simulink model "vertical_smm_with_lqr_2d"  (R2014b)
settings: Solver=FixedStepDiscrete  StartTime=0.0  StopTime=inf  FixedStep=sample_time  RelTol=1e-3
values from neighbouring files (symbols this model uses):
  forward_dx = [-0.304875592207 -0.274388032987 -0.243900473766 -0.213412914545 -0.182925355324 -0.152437796104 -0.121950236883 -0.0914626776622 -0.0609751184415 -0.0304875592207 0 0.0304875592207 ... (714 elements, 21x34)]    [ref_trajs.mat]
  forward_dx_of_dxstar = [-1.3048755994 -1.25487559904 -1.20487559868 -1.15487559832 -1.10487559796 -1.0548755976 -1.00487559724 -0.954875596883 -0.904875596523 -0.854875596164 -0.804875595804 -0.754875595707 ... (29274 elements, 41x21x34)]    [ref_trajs.mat]
  forward_x = [0.0961104217981 0.0864993796183 0.0768883374385 0.0672772952586 0.0576662530788 0.048055210899 0.0384441687192 0.0288331265394 0.0192220843596 0.00961104217981 0 -0.00961104217981 ... (714 elements, 21x34)]    [ref_trajs.mat]
  forward_x_of_dxstar = [0.247353819189 0.239791649319 0.232229479449 0.22466730958 0.21710513971 0.209542969841 0.201980799971 0.194418630102 0.186856460232 0.179294290363 0.171732120493 0.164169950675 ... (29274 elements, 41x21x34)]    [ref_trajs.mat]
  target_dx_range = [-1 -0.95 -0.9 -0.85 -0.8 -0.75 -0.7 -0.65 -0.6 -0.55 -0.5 -0.45 ... (41 elements, 1x41)]    [ref_trajs.mat]
undefined symbols (not defined in the file or in its folder): A_kalman_fourbar_gear, A_kalman_transverse, A_kalman_vertical, A_lpf_dtau, A_lpf_leg_spring, B1_lpf_dtau, B1_lpf_leg_spring, B2_lpf_dtau, B2_lpf_leg_spring, B_dx_versus_x0, B_kalman_fourbar_gear, B_kalman_transverse, B_kalman_vertical, backwards_K_sag_of_t, boom_mount_angle, C_kalman_fourbar_gear, C_kalman_transverse, C_kalman_vertical, com_leg_motor, com_torso, contact_threshold, control_start_time, d_vertical_boom_com_offset, d_vertical_com, desired_com_forward_velocity, desired_torso_angle, Discrete, fcut_contact, forward_velocity_target_step, g, h_boom, HIP_MTR_MAX_CONT_TORQUE, i_robot, initial_dx_estimate, initial_dy_estimate, initial_dz_estimate, initial_z_estimate, j_leg, j_motor, j_segments, k_LQR_vertical, k_sea, k_vertical_winch, kalman_load_to_deflect_transmission, kalman_stance_slip_threshold, kd_lateral, kd_motor, kp_lateral, kp_motor, l_boom_projected, l_retract_delta, l_retract_swing_max, l_retract_swing_min, l_seg, lambda1, lambda2, lateral_offset, lateral_target_angle_right, lateral_transition_force, left_leg_flight_y_target ... (+55)
libraries: simulink x9, ctrlSharedLib x7
(part 3 of 4)

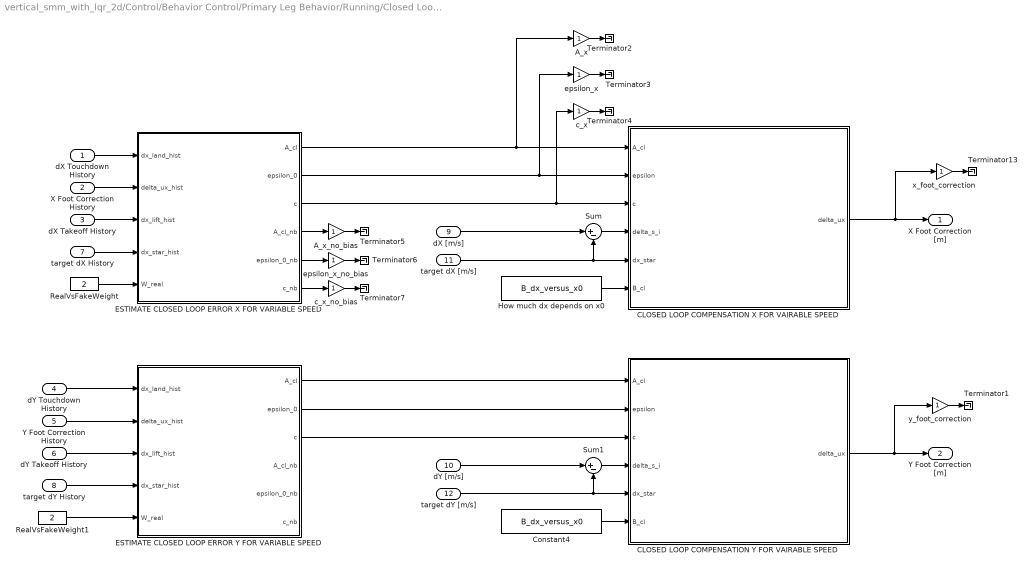
== system vertical_smm_with_lqr_2d/Control/Behavior Control/Primary Leg Behavior/Running/Closed Loop Compensation ==
  dX Touchdown History : Inport
  X Foot Correction History : Inport  Port=2
  dX Takeoff History : Inport  Port=3
  dY Touchdown History : Inport  Port=4
  Y Foot Correction History : Inport  Port=5
  dY Takeoff History : Inport  Port=6
  target dX History : Inport  Port=7
  target dY History : Inport  Port=8
  dX [m/s] : Inport  Port=9
  dY [m/s] : Inport  Port=10
  target dX [m/s] : Inport  Port=11
  "target dY [m/s] " : Inport  Port=12
  A_x : Gain
  A_x_no_bias : Gain
  CLOSED LOOP COMPENSATION X FOR VAIRABLE SPEED : MATLAB Function  TreatAsAtomicUnit=on
  CLOSED LOOP COMPENSATION Y FOR VAIRABLE SPEED : MATLAB Function  TreatAsAtomicUnit=on
  Constant4 : Constant  Value=B_dx_versus_x0
  ESTIMATE CLOSED LOOP ERROR X FOR VARIABLE SPEED : MATLAB Function  TreatAsAtomicUnit=on
  ESTIMATE CLOSED LOOP ERROR Y FOR VARIABLE SPEED : MATLAB Function  TreatAsAtomicUnit=on
  How much dx depends on x0 : Constant  Value=B_dx_versus_x0
  RealVsFakeWeight : Constant  Value=2
  RealVsFakeWeight1 : Constant  Value=2
  Sum : Sum  Inputs=|+-
  Sum1 : Sum  Inputs=|+-
  Terminator{1..7,13} (8 alike) : Terminator
  c_x : Gain
  c_x_no_bias : Gain
  epsilon_x : Gain
  epsilon_x_no_bias : Gain
  x_foot_correction : Gain
  y_foot_correction : Gain
  X Foot Correction [m] : Outport
  Y Foot Correction [m] : Outport  Port=2
  wires:
  RealVsFakeWeight1/1 -> ESTIMATE CLOSED LOOP ERROR Y FOR VARIABLE SPEED/5(W_real)
  Constant4/1 -> CLOSED LOOP COMPENSATION Y FOR VAIRABLE SPEED/6(B_cl)
  "target dY [m/s] "/1 -> Sum1/2, CLOSED LOOP COMPENSATION Y FOR VAIRABLE SPEED/5(dx_star)
  ESTIMATE CLOSED LOOP ERROR Y FOR VARIABLE SPEED/3(c) -> CLOSED LOOP COMPENSATION Y FOR VAIRABLE SPEED/3(c)
  ESTIMATE CLOSED LOOP ERROR Y FOR VARIABLE SPEED/2(epsilon_0) -> CLOSED LOOP COMPENSATION Y FOR VAIRABLE SPEED/2(epsilon)
  ESTIMATE CLOSED LOOP ERROR Y FOR VARIABLE SPEED/1(A_cl) -> CLOSED LOOP COMPENSATION Y FOR VAIRABLE SPEED/1(A_cl)
  target dY History/1 -> ESTIMATE CLOSED LOOP ERROR Y FOR VARIABLE SPEED/4(dx_star_hist)
  Y Foot Correction History/1 -> ESTIMATE CLOSED LOOP ERROR Y FOR VARIABLE SPEED/2(delta_ux_hist)
  dY Takeoff History/1 -> ESTIMATE CLOSED LOOP ERROR Y FOR VARIABLE SPEED/3(dx_lift_hist)
  dY [m/s]/1 -> Sum1/1
  RealVsFakeWeight/1 -> ESTIMATE CLOSED LOOP ERROR X FOR VARIABLE SPEED/5(W_real)
  How much dx depends on x0/1 -> CLOSED LOOP COMPENSATION X FOR VAIRABLE SPEED/6(B_cl)
  Sum/1 -> CLOSED LOOP COMPENSATION X FOR VAIRABLE SPEED/4(delta_s_i)
  target dX [m/s]/1 -> Sum/2, CLOSED LOOP COMPENSATION X FOR VAIRABLE SPEED/5(dx_star)
  ESTIMATE CLOSED LOOP ERROR X FOR VARIABLE SPEED/3(c) -> CLOSED LOOP COMPENSATION X FOR VAIRABLE SPEED/3(c), c_x/1
  ESTIMATE CLOSED LOOP ERROR X FOR VARIABLE SPEED/2(epsilon_0) -> CLOSED LOOP COMPENSATION X FOR VAIRABLE SPEED/2(epsilon), epsilon_x/1
  ESTIMATE CLOSED LOOP ERROR X FOR VARIABLE SPEED/1(A_cl) -> CLOSED LOOP COMPENSATION X FOR VAIRABLE SPEED/1(A_cl), A_x/1
  target dX History/1 -> ESTIMATE CLOSED LOOP ERROR X FOR VARIABLE SPEED/4(dx_star_hist)
  X Foot Correction History/1 -> ESTIMATE CLOSED LOOP ERROR X FOR VARIABLE SPEED/2(delta_ux_hist)
  dX Takeoff History/1 -> ESTIMATE CLOSED LOOP ERROR X FOR VARIABLE SPEED/3(dx_lift_hist)
  dX Touchdown History/1 -> ESTIMATE CLOSED LOOP ERROR X FOR VARIABLE SPEED/1(dx_land_hist)
  dX [m/s]/1 -> Sum/1
  dY Touchdown History/1 -> ESTIMATE CLOSED LOOP ERROR Y FOR VARIABLE SPEED/1(dx_land_hist)
  Sum1/1 -> CLOSED LOOP COMPENSATION Y FOR VAIRABLE SPEED/4(delta_s_i)
  CLOSED LOOP COMPENSATION X FOR VAIRABLE SPEED/1(delta_ux) -> x_foot_correction/1, X Foot Correction [m]/1
  x_foot_correction/1 -> Terminator13/1
  CLOSED LOOP COMPENSATION Y FOR VAIRABLE SPEED/1(delta_ux) -> y_foot_correction/1, Y Foot Correction [m]/1
  y_foot_correction/1 -> Terminator1/1
  A_x/1 -> Terminator2/1
  epsilon_x/1 -> Terminator3/1
  c_x/1 -> Terminator4/1
  ESTIMATE CLOSED LOOP ERROR X FOR VARIABLE SPEED/6(c_nb) -> c_x_no_bias/1
  ESTIMATE CLOSED LOOP ERROR X FOR VARIABLE SPEED/5(epsilon_0_nb) -> epsilon_x_no_bias/1
  ESTIMATE CLOSED LOOP ERROR X FOR VARIABLE SPEED/4(A_cl_nb) -> A_x_no_bias/1
  A_x_no_bias/1 -> Terminator5/1
  epsilon_x_no_bias/1 -> Terminator6/1
  c_x_no_bias/1 -> Terminator7/1

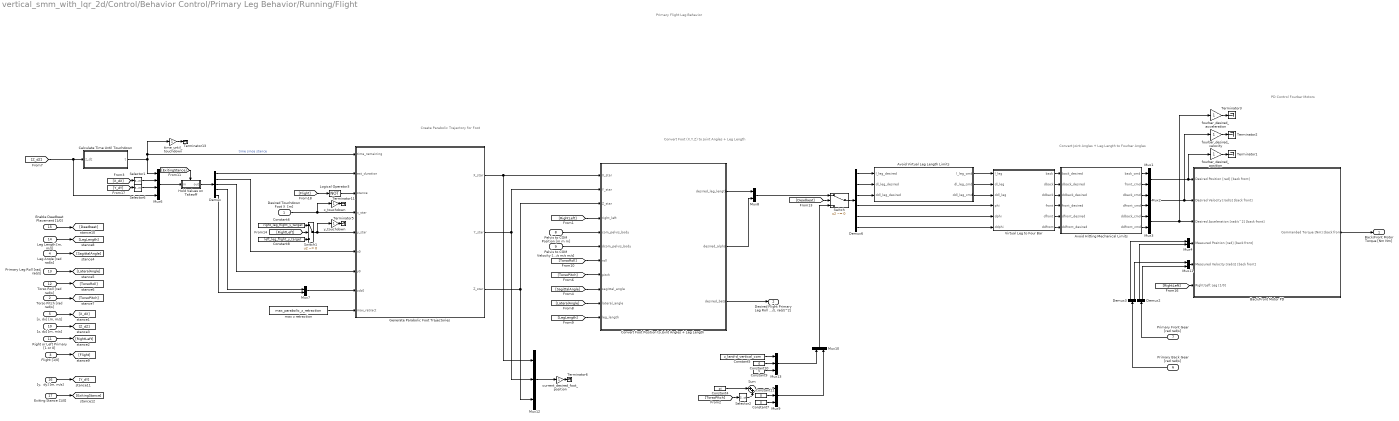
== system vertical_smm_with_lqr_2d/Control/Behavior Control/Primary Leg Behavior/Running/Flight ==
  note: Primary Flight Leg Behavior
  note: Create Parabolic
      | Trajectory for Foot
  note: Convert Foot (X,Y,Z) to
      | Joint Angles + Leg Length
  note: Convert Joint Angles + Leg Length
      | to Fourbar Angles
  note: PD Control Fourbar Motors
  Desired Touchdown Foot X  [m] : Inport
  Torso Pitch [rad rad/s] : Inport  Port=2
  Flight [1/0] : Inport  Port=3
  Leg Angle [rad rad/s] : Inport  Port=4
  "[x, dx] [m, m/s]" : Inport  Port=5
  Primary Back Gear [rad rad/s] : Inport  Port=6
  Primary Front Gear [rad rad/s] : Inport  Port=7
  Pelvis to COM Position [m m m] : Inport  Port=8
  Pelvis to COM Velocity [m/s m/s m/s] : Inport  Port=9
  "[z, dz] [m, m/s]" : Inport  Port=10
  Right or Left Primary [1 or 0] : Inport  Port=11
  Torso Roll [rad rad/s] : Inport  Port=12
  "Primary Leg Roll [rad, rad/s]" : Inport  Port=13
  "Leg Length [m, m/s]" : Inport  Port=14
  Enable Deadbeat Placement [1/0] : Inport  Port=15
  "[y,  dy] [m, m/s]" : Inport  Port=16
  Exiting Stance [1/0] : Inport  Port=17
  Avoid Hitting Mechanical Limits : MATLAB Function  TreatAsAtomicUnit=on
  Avoid Virtual Leg Length Limits : MATLAB Function  TreatAsAtomicUnit=on
  Back/Front Motor PD : Subsystem
  Calculate Time Until Touchdown : MATLAB Function  TreatAsAtomicUnit=on
  Constant{7,9..11} (4 alike) : Constant  Value=0
  Constant4 : Constant  Value=pi
  Constant5 : Constant  Value=z_land-d_vertical_com
  Constant6 : Constant  Value=right_leg_flight_y_target
  Constant8 : Constant  Value=left_leg_flight_y_target
  "Convert Foot Position to Joint Angles + Leg Length " : MATLAB Function  TreatAsAtomicUnit=on
  Demux : Demux  Outputs=5
  Demux2 : Demux  Outputs=2
  Demux3 : Demux  Outputs=2
  Demux6 : Demux  Outputs=6
  Generate Parabolic Foot Trajectories : MATLAB Function  TreatAsAtomicUnit=on
  Hold Values on Takeoff : Subsystem
  Logical Operator3 : Logic  Operator=NOT  AllPortsSameDT=off  OutDataTypeStr=boolean
  Mux{1..4,7..8,10..11} (8 alike) : Mux  Inputs=2
  Mux12 : Mux  Inputs=3
  Mux13 : Mux  Inputs=3
  Mux6 : Mux
  Mux9 : Mux  Inputs=3
  Selector1 : Selector  InputPortWidth=2  Indices=[1]
  Selector2 : Selector  InputPortWidth=2  Indices=[1]
  Selector6 : Selector  InputPortWidth=2  Indices=[1]
  Sum : Sum  Inputs=|++
  Switch : Switch  Criteria=u2 ~= 0
  Switch1 : Switch  Criteria=u2 ~= 0
  Terminator{1..3,5..6,11,13} (7 alike) : Terminator
  Virtual Leg to Four Bar : MATLAB Function  TreatAsAtomicUnit=on
  current_desired_foot_position : Gain
  fourbar_desired_acceleration : Gain
  fourbar_desired_position : Gain
  fourbar_desired_velocity : Gain
  max z retraction : Constant  Value=max_parabolic_z_retraction
  time_until_touchdown : Gain
  x_touchdown : Gain
  y_touchdown : Gain
  Back/Front Motor Torque [Nm Nm] : Outport
  "Desired Flight Primary Leg Roll [rad, rad/s, rad/s^2]" : Outport  Port=2
  wires:
  Virtual Leg to Four Bar/1(back) -> Avoid Hitting Mechanical Limits/1(back_desired)
  Virtual Leg to Four Bar/2(dback) -> Avoid Hitting Mechanical Limits/2(dback_desired)
  Virtual Leg to Four Bar/3(ddback) -> Avoid Hitting Mechanical Limits/3(ddback_desired)
  Virtual Leg to Four Bar/4(front) -> Avoid Hitting Mechanical Limits/4(front_desired)
  Virtual Leg to Four Bar/5(dfront) -> Avoid Hitting Mechanical Limits/5(dfront_desired)
  Virtual Leg to Four Bar/6(ddfront) -> Avoid Hitting Mechanical Limits/6(ddfront_desired)
  Mux11/1 -> Back/Front Motor PD/5(Measured Velocity [rad/s] [back front])
  Demux2/2 -> Mux11/2
  Mux4/1 -> Back/Front Motor PD/4(Measured Position [rad] [back front])
  Mux1/1 -> fourbar_desired_position/1, Back/Front Motor PD/1(Desired Position [rad] [back front])
  Demux3/2 -> Mux11/1
  Demux3/1 -> Mux4/1
  Avoid Hitting Mechanical Limits/2(front_cmd) -> Mux1/2
  Avoid Hitting Mechanical Limits/1(back_cmd) -> Mux1/1
  Demux2/1 -> Mux4/2
  Avoid Hitting Mechanical Limits/3(dback_cmd) -> Mux2/1
  Avoid Hitting Mechanical Limits/4(dfront_cmd) -> Mux2/2
  Avoid Hitting Mechanical Limits/5(ddback_cmd) -> Mux3/1
  Avoid Hitting Mechanical Limits/6(ddfront_cmd) -> Mux3/2
  Mux2/1 -> fourbar_desired_velocity/1, Back/Front Motor PD/2(Desired Velocity [rad/s] [back front])
  Mux3/1 -> fourbar_desired_acceleration/1, Back/Front Motor PD/3(Desired Acceleration [rad/s^2] [back front])
  Back/Front Motor PD/1(Commanded Torque [Nm] [back front]) -> Back/Front Motor Torque [Nm Nm]/1
  Primary Back Gear [rad rad/s]/1 -> Demux3/1
  Primary Front Gear [rad rad/s]/1 -> Demux2/1
  [RightLeft] -> Back/Front Motor PD/6(Right/Left Leg [1/0])
  fourbar_desired_position/1 -> Terminator1/1
  fourbar_desired_velocity/1 -> Terminator2/1
  fourbar_desired_acceleration/1 -> Terminator3/1
  Demux/1 -> Generate Parabolic Foot Trajectories/2(est_duration)
  Mux7/1 -> Generate Parabolic Foot Trajectories/8(zdz0)
  max z retraction/1 -> Generate Parabolic Foot Trajectories/9(max_retract)
  Logical Operator3/1 -> Generate Parabolic Foot Trajectories/3(stance)
  Mux6/1 -> Hold Values on Takeoff/1(in)
  Hold Values on Takeoff/1(out) -> Demux/1
  Switch1/1 -> Generate Parabolic Foot Trajectories/5(y_star), y_touchdown/1
  Selector1/1 -> Mux6/2
  [X_dX] -> Selector1/1
  Generate Parabolic Foot Trajectories/1(X_star) -> "Convert Foot Position to Joint Angles + Leg Length "/1(X_star), Mux12/1
  Generate Parabolic Foot Trajectories/2(Y_star) -> "Convert Foot Position to Joint Angles + Leg Length "/2(Y_star), Mux12/2
  Generate Parabolic Foot Trajectories/3(Z_star) -> "Convert Foot Position to Joint Angles + Leg Length "/3(Z_star), Mux12/3
  [RightLeft] -> "Convert Foot Position to Joint Angles + Leg Length "/4(right_left)
  "Convert Foot Position to Joint Angles + Leg Length "/2(desired_alpha) -> Mux8/2
  "Convert Foot Position to Joint Angles + Leg Length "/1(desired_leg_length) -> Mux8/1
  "Convert Foot Position to Joint Angles + Leg Length "/3(desired_beta) -> "Desired Flight Primary Leg Roll [rad, rad/s, rad/s^2]"/1
  Demux6/6 -> Virtual Leg to Four Bar/6(ddphi)
  Demux6/5 -> Virtual Leg to Four Bar/5(dphi)
  Demux6/4 -> Virtual Leg to Four Bar/4(phi)
  Switch/1 -> Demux6/1
  Mux8/1 -> Switch/1
  Constant7/1 -> Mux9/3
  Mux10/1 -> Switch/3
  Mux9/1 -> Mux10/2
  Leg Angle [rad rad/s]/1 -> [SagittalAngle]
  [SagittalAngle] -> "Convert Foot Position to Joint Angles + Leg Length "/9(sagittal_angle)
  Torso Pitch [rad rad/s]/1 -> [TorsoPitch]
  [TorsoPitch] -> "Convert Foot Position to Joint Angles + Leg Length "/8(pitch)
  [LateralAngle] -> "Convert Foot Position to Joint Angles + Leg Length "/10(lateral_angle)
  [LegLength] -> "Convert Foot Position to Joint Angles + Leg Length "/11(leg_length)
  [TorsoRoll] -> "Convert Foot Position to Joint Angles + Leg Length "/7(roll)
  Pelvis to COM Position [m m m]/1 -> "Convert Foot Position to Joint Angles + Leg Length "/5(com_pelvis_body)
  Pelvis to COM Velocity [m/s m/s m/s]/1 -> "Convert Foot Position to Joint Angles + Leg Length "/6(dcom_pelvis_body)
  Flight [1/0]/1 -> [Flight]
  [ExitingStance] -> Hold Values on Takeoff/Trigger
  [Deadbeat] -> Switch/2
  [RightLeft] -> Switch1/2
  Constant6/1 -> Switch1/1
  Constant8/1 -> Switch1/3
  "[x, dx] [m, m/s]"/1 -> [X_dX]
  Right or Left Primary [1 or 0]/1 -> [RightLeft]
  Torso Roll [rad rad/s]/1 -> [TorsoRoll]
  "Primary Leg Roll [rad, rad/s]"/1 -> [LateralAngle]
  "Leg Length [m, m/s]"/1 -> [LegLength]
  Enable Deadbeat Placement [1/0]/1 -> [Deadbeat]
  "[z, dz] [m, m/s]"/1 -> [Z_dZ]
  Desired Touchdown Foot X  [m]/1 -> x_touchdown/1, Generate Parabolic Foot Trajectories/4(x_star)
  x_touchdown/1 -> Terminator11/1
  y_touchdown/1 -> Terminator5/1
  current_desired_foot_position/1 -> Terminator6/1
  Mux12/1 -> current_desired_foot_position/1
  "[y,  dy] [m, m/s]"/1 -> [Y_dY]
  [Y_dY] -> Selector6/1
  [Z_dZ] -> Mux6/4, Calculate Time Until Touchdown/1(z_dz)
  Selector6/1 -> Mux6/3
  Demux/2 -> Generate Parabolic Foot Trajectories/6(x0)
  Demux/3 -> Generate Parabolic Foot Trajectories/7(y0)
  Demux/4 -> Mux7/1
  Demux/5 -> Mux7/2
  Calculate Time Until Touchdown/1(t) -> Mux6/1, time_until_touchdown/1, Generate Parabolic Foot Trajectories/1(time_remaining)  "time since stance"
  time_until_touchdown/1 -> Terminator13/1
  [Flight] -> Logical Operator3/1
  Constant11/1 -> Mux9/2
  Sum/1 -> Mux9/1
  Constant5/1 -> Mux13/1
  Constant9/1 -> Mux13/3
  Constant10/1 -> Mux13/2
  Mux13/1 -> Mux10/1
  Avoid Virtual Leg Length Limits/1(l_leg_cmd) -> Virtual Leg to Four Bar/1(l_leg)
  Avoid Virtual Leg Length Limits/2(dl_leg_cmd) -> Virtual Leg to Four Bar/2(dl_leg)
  Avoid Virtual Leg Length Limits/3(ddl_leg_cmd) -> Virtual Leg to Four Bar/3(ddl_leg)
  Demux6/1 -> Avoid Virtual Leg Length Limits/1(l_leg_desired)
  Demux6/2 -> Avoid Virtual Leg Length Limits/2(dl_leg_desired)
  Demux6/3 -> Avoid Virtual Leg Length Limits/3(ddl_leg_desired)
  Constant4/1 -> Sum/1
  [TorsoPitch] -> Selector2/1
  Selector2/1 -> Sum/2
  Exiting Stance [1/0]/1 -> [ExitingStance]

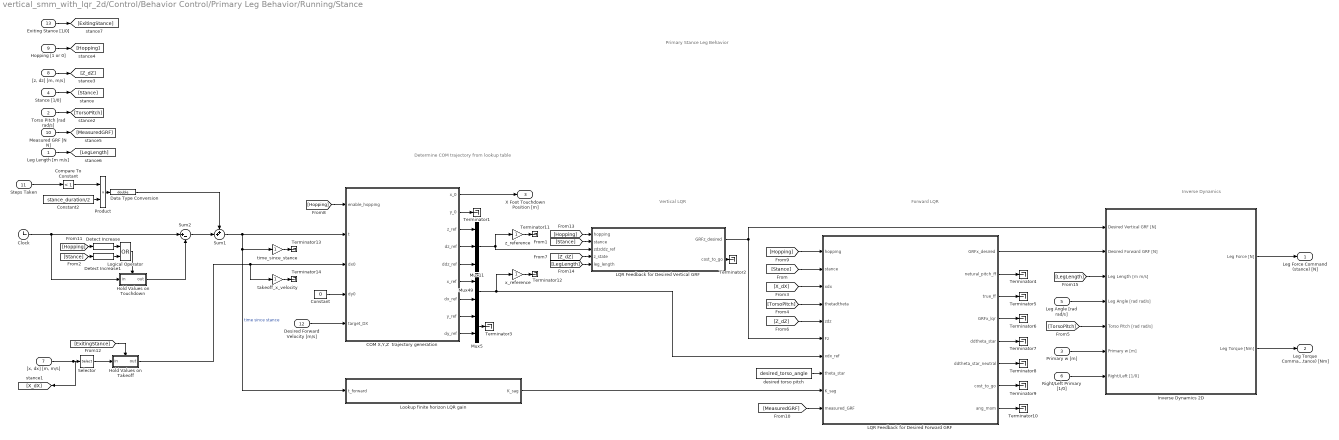
== system vertical_smm_with_lqr_2d/Control/Behavior Control/Primary Leg Behavior/Running/Stance ==
  note: Primary Stance Leg Behavior
  note: Determine COM trajectory
      | from lookup table
  note: Vertical LQR
  note: Forward LQR
  note: Inverse Dynamics
  Leg Length [m m/s] : Inport
  Torso Pitch [rad rad/s] : Inport  Port=2
  Primary w [m] : Inport  Port=3
  Stance [1/0] : Inport  Port=4
  Leg Angle [rad rad/s] : Inport  Port=5
  Right/Left Primary [1/0] : Inport  Port=6
  "[x, dx] [m, m/s]" : Inport  Port=7
  "[z, dz] [m, m/s]" : Inport  Port=8
  Hopping [1 or 0] : Inport  Port=9
  Measured GRF [N N] : Inport  Port=10
  Steps Taken : Inport  Port=11
  Desired Forward Velocity [m/s] : Inport  Port=12
  Exiting Stance [1/0] : Inport  Port=13
  COM X,Y,Z  trajectory generation : MATLAB Function  TreatAsAtomicUnit=on
  Clock : Clock
  Compare To Constant : simulink/Logic and Bit Operations/Compare To Constant  relop=<  const=1  OutDataTypeStr=uint8
  Constant : Constant  Value=0
  Constant2 : Constant  Value=stance_duration/2
  Data Type Conversion : DataTypeConversion  OutDataTypeStr=double
  Detect Increase : simulink/Logic and Bit Operations/Detect Increase  vinit=0.0  InputProcessing=Inherited  OutDataTypeStr=boolean
  Detect Increase1 : simulink/Logic and Bit Operations/Detect Increase  vinit=0.0  InputProcessing=Inherited  OutDataTypeStr=boolean
  Hold Values on Takeoff : Subsystem
  Hold Values on Touchdown : Subsystem
  Inverse Dynamics 2D : Subsystem
  LQR Feedback for Desired Forward GRF : MATLAB Function  TreatAsAtomicUnit=on
  LQR Feedback for Desired Vertical GRF : MATLAB Function  TreatAsAtomicUnit=on
  Logical Operator : Logic  Operator=OR  AllPortsSameDT=off  OutDataTypeStr=boolean
  Lookup finite horizon LQR gain : MATLAB Function  TreatAsAtomicUnit=on
  Mux11 : Mux  Inputs=3
  Mux49 : Mux  Inputs=2
  Mux5 : Mux  Inputs=2
  Product : Product
  Selector : Selector  InputPortWidth=2  Indices=[2]
  Sum1 : Sum  Inputs=++|  OutDataTypeStr=double
  Sum2 : Sum  Inputs=|+-
  Terminator{1..14} (14 alike) : Terminator
  desired torso pitch : Constant  Value=desired_torso_angle
  takeoff_x_velocity : Gain
  time_since_stance : Gain
  x_reference : Gain
  z_reference : Gain
  Leg Force Command (stance) [N] : Outport
  Leg Torque Command (stance) [Nm] : Outport  Port=2
  X Foot Touchdown Position [m] : Outport  Port=3
  wires:
  Inverse Dynamics 2D/2(Leg Torque [Nm]) -> Leg Torque Command (stance) [Nm]/1
  Inverse Dynamics 2D/1(Leg Force [N]) -> Leg Force Command (stance) [N]/1
  Mux5/1 -> Terminator3/1
  [Z_dZ] -> LQR Feedback for Desired Vertical GRF/4(z_state)
  COM X,Y,Z  trajectory generation/3(z_ref) -> Mux11/1
  [Stance] -> LQR Feedback for Desired Forward GRF/2(stance)
  COM X,Y,Z  trajectory generation/6(x_ref) -> Mux49/1
  COM X,Y,Z  trajectory generation/7(dx_ref) -> Mux49/2
  COM X,Y,Z  trajectory generation/8(y_ref) -> Mux5/1
  COM X,Y,Z  trajectory generation/9(dy_ref) -> Mux5/2
  COM X,Y,Z  trajectory generation/1(x_0) -> X Foot Touchdown Position [m]/1
  COM X,Y,Z  trajectory generation/4(dz_ref) -> Mux11/2
  COM X,Y,Z  trajectory generation/5(ddz_ref) -> Mux11/3
  Mux11/1 -> z_reference/1, LQR Feedback for Desired Vertical GRF/3(zdzddz_ref)
  [X_dX] -> LQR Feedback for Desired Forward GRF/3(xdx)
  [TorsoPitch] -> LQR Feedback for Desired Forward GRF/4(thetadtheta)
  Mux49/1 -> x_reference/1, LQR Feedback for Desired Forward GRF/7(xdx_ref)
  desired torso pitch/1 -> LQR Feedback for Desired Forward GRF/8(theta_star)
  Lookup finite horizon LQR gain/1(K_sag) -> LQR Feedback for Desired Forward GRF/9(K_sag)
  [Z_dZ] -> LQR Feedback for Desired Forward GRF/5(zdz)
  Desired Forward Velocity [m/s]/1 -> COM X,Y,Z  trajectory generation/5(target_DX)
  LQR Feedback for Desired Forward GRF/1(GRFx_desired) -> Inverse Dynamics 2D/2(Desired Forward GRF [N])
  Sum1/1 -> time_since_stance/1, Lookup finite horizon LQR gain/1(t_forward), COM X,Y,Z  trajectory generation/2(t)  "time since stance"
  LQR Feedback for Desired Vertical GRF/1(GRFz_desired) -> Inverse Dynamics 2D/1(Desired Vertical GRF [N]), LQR Feedback for Desired Forward GRF/6(Fz)
  Hold Values on Touchdown/1(out) -> Sum2/2
  Stance [1/0]/1 -> [Stance]
  [Stance] -> LQR Feedback for Desired Vertical GRF/2(stance)
  Logical Operator/1 -> Hold Values on Touchdown/Trigger
  "[x, dx] [m, m/s]"/1 -> [X_dX], Selector/1
  Clock/1 -> Hold Values on Touchdown/1(in), Sum2/1
  Constant/1 -> COM X,Y,Z  trajectory generation/4(dy0)
  LQR Feedback for Desired Vertical GRF/2(cost_to_go) -> Terminator2/1
  LQR Feedback for Desired Forward GRF/2(netural_pitch_ff) -> Terminator4/1
  LQR Feedback for Desired Forward GRF/3(true_ff) -> Terminator5/1
  LQR Feedback for Desired Forward GRF/4(GRFx_lqr) -> Terminator6/1
  LQR Feedback for Desired Forward GRF/5(ddtheta_star) -> Terminator7/1
  LQR Feedback for Desired Forward GRF/6(ddtheta_star_neutral) -> Terminator8/1
  LQR Feedback for Desired Forward GRF/7(cost_to_go) -> Terminator9/1
  LQR Feedback for Desired Forward GRF/8(ang_mom) -> Terminator10/1
  [LegLength] -> Inverse Dynamics 2D/3(Leg Length [m m/s])
  Leg Angle [rad rad/s]/1 -> Inverse Dynamics 2D/4(Leg Angle [rad rad/s])
  Torso Pitch [rad rad/s]/1 -> [TorsoPitch]
  [TorsoPitch] -> Inverse Dynamics 2D/5(Torso Pitch [rad rad/s])
  Primary w [m]/1 -> Inverse Dynamics 2D/6(Primary w [m])
  Right/Left Primary [1/0]/1 -> Inverse Dynamics 2D/7(Right/Left [1/0])
  "[z, dz] [m, m/s]"/1 -> [Z_dZ]
  COM X,Y,Z  trajectory generation/2(y_0) -> Terminator1/1
  Hopping [1 or 0]/1 -> [Hopping]
  [Hopping] -> COM X,Y,Z  trajectory generation/1(enable_hopping)
  z_reference/1 -> Terminator11/1
  x_reference/1 -> Terminator12/1
  [Hopping] -> LQR Feedback for Desired Forward GRF/1(hopping)
  Measured GRF [N N]/1 -> [MeasuredGRF]
  [MeasuredGRF] -> LQR Feedback for Desired Forward GRF/10(measured_GRF)
  Steps Taken/1 -> Compare To Constant/1
  Product/1 -> Data Type Conversion/1
  Constant2/1 -> Product/2
  Detect Increase/1 -> Logical Operator/1
  Detect Increase1/1 -> Logical Operator/2
  Compare To Constant/1 -> Product/1
  Sum2/1 -> Sum1/2
  Data Type Conversion/1 -> Sum1/1
  time_since_stance/1 -> Terminator13/1
  [Hopping] -> Detect Increase/1
  [Stance] -> Detect Increase1/1
  Hold Values on Takeoff/1(out) -> takeoff_x_velocity/1, COM X,Y,Z  trajectory generation/3(dx0)
  [ExitingStance] -> Hold Values on Takeoff/Trigger
  takeoff_x_velocity/1 -> Terminator14/1
  Selector/1 -> Hold Values on Takeoff/1(in)
  [Hopping] -> LQR Feedback for Desired Vertical GRF/1(hopping)
  [LegLength] -> LQR Feedback for Desired Vertical GRF/5(leg_length)
  Leg Length [m m/s]/1 -> [LegLength]
  Exiting Stance [1/0]/1 -> [ExitingStance]

== system vertical_smm_with_lqr_2d/Control/Behavior Control/Secondary Leg Behavior/Back//Front Motor PD/Friction Compensation ==
  Right/Left [1/0] : Inport
  Commanded Velocity [rad/s] [back front] : Inport  Port=2
  Product : Product
  Sign : Signum
  Sum1 : Sum
  Switch : Switch  Criteria=u2 ~= 0
  Switch1 : Switch  Criteria=u2 ~= 0
  coulomb_friction_left : Constant  Value=sea_coulomb_friction(3:4)
  coulomb_friction_right : Constant  Value=sea_coulomb_friction(1:2)
  offset_friction_left : Constant  Value=sea_offset_friction(3:4)
  offset_friction_right : Constant  Value=sea_offset_friction(1:2)
  Friction Compensation [Nm] : Outport
  wires:
  Commanded Velocity [rad/s] [back front]/1 -> Sign/1
  Switch/1 -> Sum1/2
  Sum1/1 -> Friction Compensation [Nm]/1
  Product/1 -> Sum1/1
  Right/Left [1/0]/1 -> Switch1/2, Switch/2
  offset_friction_right/1 -> Switch/1
  offset_friction_left/1 -> Switch/3
  coulomb_friction_right/1 -> Switch1/1
  coulomb_friction_left/1 -> Switch1/3
  Switch1/1 -> Product/2
  Sign/1 -> Product/1

== system vertical_smm_with_lqr_2d/Control/Behavior Control/Primary Leg Behavior/Running/Circular Buffer/Enabled on Touchdown ==
  In : Inport
  Enable : EnablePort
  Out : Outport
  wires:
  In/1 -> Out/1

== system vertical_smm_with_lqr_2d/Control/Behavior Control/Primary Leg Behavior/Running/Flight/Back//Front Motor PD ==
  Desired Position [rad] [back front] : Inport
  Desired Velocity [rad/s] [back front] : Inport  Port=2
  Desired Acceleration [rad/s^2] [back front] : Inport  Port=3
  Measured Position [rad] [back front] : Inport  Port=4
  Measured Velocity [rad/s] [back front] : Inport  Port=5
  Right/Left Leg [1/0] : Inport  Port=6
  Friction Compensation : Subsystem
  Product : Product
  Sum1 : Sum  Inputs=|++
  Sum2 : Sum  Inputs=|++
  Sum7 : Sum  Inputs=|+-
  Sum8 : Sum  Inputs=|+-
  Sum9 : Sum
  kd : Gain  Gain=kd_motor
  kp : Gain  Gain=kp_motor
  reflected inertia : Constant  Value=j_motor
  Commanded Torque [Nm] [back front] : Outport
  wires:
  kp/1 -> Sum9/1
  Sum7/1 -> kp/1
  Measured Position [rad] [back front]/1 -> Sum7/2
  Sum9/1 -> Sum1/1
  Sum8/1 -> kd/1
  Desired Position [rad] [back front]/1 -> Sum7/1
  kd/1 -> Sum9/2
  Measured Velocity [rad/s] [back front]/1 -> Sum8/2
  Sum1/1 -> Sum2/1
  Desired Acceleration [rad/s^2] [back front]/1 -> Product/1
  Product/1 -> Sum1/2
  Right/Left Leg [1/0]/1 -> Friction Compensation/1(Right/Left [1/0])
  Sum2/1 -> Commanded Torque [Nm] [back front]/1
  Desired Velocity [rad/s] [back front]/1 -> Friction Compensation/2(Commanded Velocity [rad/s] [back front]), Sum8/1
  reflected inertia/1 -> Product/2
  Friction Compensation/1(Friction Compensation [Nm]) -> Sum2/2

== system vertical_smm_with_lqr_2d/Control/Behavior Control/Primary Leg Behavior/Running/Flight/Hold Values on Takeoff ==
  in : Inport
  Trigger : TriggerPort  ShowOutputPort=on  PortDimensions=1
  Subsystem : Subsystem
  out : Outport
  wires:
  Trigger/1 -> Subsystem/Enable
  Subsystem/1(out) -> out/1
  in/1 -> Subsystem/1(in)

== system vertical_smm_with_lqr_2d/Control/Behavior Control/Primary Leg Behavior/Running/Stance/Hold Values on Takeoff ==
  in : Inport
  Trigger : TriggerPort  ShowOutputPort=on  PortDimensions=1
  Subsystem : Subsystem
  out : Outport
  wires:
  Trigger/1 -> Subsystem/Enable
  Subsystem/1(out) -> out/1
  in/1 -> Subsystem/1(in)

== system vertical_smm_with_lqr_2d/Control/Behavior Control/Primary Leg Behavior/Running/Stance/Hold Values on Touchdown ==
  in : Inport
  Trigger : TriggerPort  ShowOutputPort=on  PortDimensions=1
  Subsystem : Subsystem
  out : Outport
  wires:
  in/1 -> Subsystem/1(in)
  Subsystem/1(out) -> out/1
  Trigger/1 -> Subsystem/Enable

== system vertical_smm_with_lqr_2d/Control/Behavior Control/Primary Leg Behavior/Running/Stance/Inverse Dynamics 2D ==
  Desired Vertical GRF [N] : Inport
  Desired Forward GRF [N] : Inport  Port=2
  Leg Length [m m/s] : Inport  Port=3
  Leg Angle [rad rad/s] : Inport  Port=4
  Torso Pitch [rad rad/s] : Inport  Port=5
  Primary w [m] : Inport  Port=6
  Right/Left [1/0] : Inport  Port=7
  Constant2 : Constant  Value=0
  Demux5 : Demux  Outputs=2
  Leg Force-Torque Distribution : Subsystem
  Spring Torques : Selector  InputPortWidth=7  Indices=[6 7]
  Terminator1 : Terminator
  Terminator3 : Terminator
  desired_forward_GRF : Gain
  desired_vertical_GRF : Gain
  target_GRF_inverse_dynamics : MATLAB Function  TreatAsAtomicUnit=on
  Leg Force [N] : Outport
  Leg Torque [Nm] : Outport  Port=2
  wires:
  Leg Force-Torque Distribution/1(Leg Force [N]) -> Leg Force [N]/1
  Leg Angle [rad rad/s]/1 -> target_GRF_inverse_dynamics/5(phi)
  Torso Pitch [rad rad/s]/1 -> target_GRF_inverse_dynamics/4(theta)
  Leg Force-Torque Distribution/2(Leg Torque [Nm]) -> Leg Torque [Nm]/1
  Primary w [m]/1 -> Leg Force-Torque Distribution/3(w [m]), target_GRF_inverse_dynamics/7(w)
  Spring Torques/1 -> Demux5/1
  Demux5/1 -> Leg Force-Torque Distribution/1(Front Spring Torque [Nm])
  Demux5/2 -> Leg Force-Torque Distribution/2(Back Spring Torque [Nm])
  target_GRF_inverse_dynamics/1(z) -> Spring Torques/1
  Constant2/1 -> target_GRF_inverse_dynamics/9(tau_rotor_b), target_GRF_inverse_dynamics/8(tau_rotor_f)
  Leg Length [m m/s]/1 -> target_GRF_inverse_dynamics/6(l_leg)
  Right/Left [1/0]/1 -> target_GRF_inverse_dynamics/3(right_left)
  Desired Forward GRF [N]/1 -> desired_forward_GRF/1, target_GRF_inverse_dynamics/1(GRFx)
  desired_forward_GRF/1 -> Terminator3/1
  Desired Vertical GRF [N]/1 -> desired_vertical_GRF/1, target_GRF_inverse_dynamics/2(GRFz)
  desired_vertical_GRF/1 -> Terminator1/1

== system vertical_smm_with_lqr_2d/Control/Behavior Control/Primary Leg Behavior/Running/Flight/Back//Front Motor PD/Friction Compensation ==
  Right/Left [1/0] : Inport
  Commanded Velocity [rad/s] [back front] : Inport  Port=2
  Product : Product
  Sign : Signum
  Sum1 : Sum
  Switch : Switch  Criteria=u2 ~= 0
  Switch1 : Switch  Criteria=u2 ~= 0
  coulomb_friction_left : Constant  Value=sea_coulomb_friction(3:4)
  coulomb_friction_right : Constant  Value=sea_coulomb_friction(1:2)
  offset_friction_left : Constant  Value=sea_offset_friction(3:4)
  offset_friction_right : Constant  Value=sea_offset_friction(1:2)
  Friction Compensation [Nm] : Outport
  wires:
  Commanded Velocity [rad/s] [back front]/1 -> Sign/1
  Switch/1 -> Sum1/2
  Sum1/1 -> Friction Compensation [Nm]/1
  Product/1 -> Sum1/1
  Right/Left [1/0]/1 -> Switch1/2, Switch/2
  offset_friction_right/1 -> Switch/1
  offset_friction_left/1 -> Switch/3
  coulomb_friction_right/1 -> Switch1/1
  coulomb_friction_left/1 -> Switch1/3
  Switch1/1 -> Product/2
  Sign/1 -> Product/1

== system vertical_smm_with_lqr_2d/Control/Behavior Control/Primary Leg Behavior/Running/Flight/Hold Values on Takeoff/Subsystem ==
  in : Inport
  Enable : EnablePort
  out : Outport
  wires:
  in/1 -> out/1

== system vertical_smm_with_lqr_2d/Control/Behavior Control/Primary Leg Behavior/Running/Stance/Hold Values on Takeoff/Subsystem ==
  in : Inport
  Enable : EnablePort
  out : Outport
  wires:
  in/1 -> out/1

== system vertical_smm_with_lqr_2d/Control/Behavior Control/Primary Leg Behavior/Running/Stance/Hold Values on Touchdown/Subsystem ==
  in : Inport
  Enable : EnablePort
  out : Outport
  wires:
  in/1 -> out/1

== system vertical_smm_with_lqr_2d/Control/Behavior Control/Primary Leg Behavior/Running/Stance/Inverse Dynamics 2D/Leg Force-Torque Distribution ==
  Front Spring Torque [Nm] : Inport
  Back Spring Torque [Nm] : Inport  Port=2
  w [m] : Inport  Port=3
  Divide : Product  Inputs=*/
  Sum2 : Sum  Inputs=+|+
  Sum5 : Sum  Inputs=+|-
  Leg Force [N] : Outport
  Leg Torque [Nm] : Outport  Port=2
  wires:
  Sum2/1 -> Leg Torque [Nm]/1
  Back Spring Torque [Nm]/1 -> Sum5/2, Sum2/2
  Sum5/1 -> Divide/1
  w [m]/1 -> Divide/2
  Front Spring Torque [Nm]/1 -> Sum5/1, Sum2/1
  Divide/1 -> Leg Force [N]/1

== stateflow chart vertical_smm_with_lqr_2d/Control/Behavior Control/Primary Leg Behavior/State Machine ==
  state TouchDown
  state LockedContact
  state Unloading
  state Takeoff
  state Flight
  (junction 91) -> TouchDown
  TouchDown -> (junction 130) [order 2] : [vertical_grf < contact_threshold]
  (junction 93) -> (junction 91)
  (junction 130) -> (junction 128)
  TouchDown -> LockedContact [order 1] : [vertical_grf > loaded_threshold]
  (junction 115) -> LockedContact
  (junction 118) -> (junction 115)
  LockedContact -> Unloading : [leg_velocity >= 0 && previous_leg_velocity < 0]
  Unloading -> LockedContact [order 2] : [vertical_grf > loaded_threshold && leg_velocity < 0]
  (junction 122) -> (junction 118)
  Unloading -> Takeoff [order 1] : [vertical_grf < contact_threshold || leg_length > max_leg_length]
  Takeoff -> Flight : after(t_flight,sec)
  (default) -> Flight
  Flight -> (junction 93) : [vertical_grf > contact_threshold]
  (junction 128) -> Flight
  data: leg_length input; leg_velocity input; previous_leg_velocity input; vertical_grf input; t_flight parameter; max_leg_length parameter; contact_threshold parameter; loaded_threshold parameter; TouchDown output boolean; LockedContact output boolean; Unloading output boolean; Takeoff output boolean; Flight output boolean

== matlab function vertical_smm_with_lqr_2d/Control/Behavior Control/Primary Leg Behavior/Running/Stance/LQR Feedback for Desired Forward GRF ==
  data: hopping input; stance input; GRFx_desired output; netural_pitch_ff output; true_ff output; GRFx_lqr output; ddtheta_star output; ddtheta_star_neutral output; xdx input; thetadtheta input; zdz input; Fz input; xdx_ref input size=2; theta_star input; K_sag input; measured_GRF input; i_robot parameter; P_LQR_sagittal parameter; cost_to_go output double size=1; ang_mom output
%% LQR for x state

% stance: 1 if in stance, 0 otherwise
% xdx: [ x from stance leg to COM, dx of COM]
% thetadtheta: [pitch, dpitch]
% zdz: [z of COM, dz of COM]
% Fz: Desired z GRF
% xdx_ref: [x, dx] current reference point for COM
% theta_star: desired torso pitch
% K_sag: time dependent LQR gain


% sagittal_state: [x, pitch, dx, dptich]
% theta_star: desired torso pitch


function [GRFx_desired, netural_pitch_ff, true_ff, GRFx_lqr, ddtheta_star, ddtheta_star_neutral, cost_to_go, ang_mom]  =  ...
    LQR_Sagittal(hopping, stance, xdx, thetadtheta, zdz, Fz, xdx_ref, theta_star, K_sag, measured_GRF, i_robot,...
    P_LQR_sagittal)

    sagittal_state = [xdx(1); thetadtheta(1); xdx(2); thetadtheta(2)];
    sagittal_reference = [xdx_ref(1), theta_star, xdx_ref(2), 0]';
    
    % make the target pitch depend on current pitch rate s.t system ends at theta_star after flight
%     sagittal_reference = [xdx_ref(1), theta_star - f_duration*thetadtheta(2), xdx_ref(2), 0]';
    sagittal_error = (sagittal_state - sagittal_reference);
    
   
    GRFx_lqr = - K_sag*sagittal_error;
    cost_to_go = sagittal_error'*P_LQR_sagittal*sagittal_error;
    netural_pitch_ff = Fz*xdx(1)/zdz(1);
    true_ff = Fz*xdx_ref(1)/zdz(1);
    
    if stance == 0
      GRFx_lqr = 0;
      cost_to_go = 0;
      netural_pitch_ff = 0;
      true_ff = 0;
    end
    
    GRFx_desired = netural_pitch_ff + GRFx_lqr;
    %GRFx_desired = i_robot/zdz(1)*(-150*(theta_star-thetadtheta(1)) + 30*thetadtheta(2)) + netural_pitch_ff;
    if ~hopping % different PD law for lowering off the winch
        GRFx_desired = i_robot/zdz(1)*(-150*(theta_star-thetadtheta(1)) + 30*thetadtheta(2)) + netural_pitch_ff;
    end
    GRFx_desired = min(max(GRFx_desired, -abs(measured_GRF(2))/2), abs(measured_GRF(2))/2); % saturate to friction cone (mu = 0.5)
       
    % quantities for logging
    ddtheta_star_neutral = -(GRFx_lqr)*zdz(1)/i_robot;
    ddtheta_star = -(GRFx_desired - netural_pitch_ff)*zdz(1)/i_robot;
    ang_mom = i_robot*thetadtheta(2);
end

== matlab function vertical_smm_with_lqr_2d/Control/Behavior Control/Torque Distribution Right/Motor Torque Saturation Optimization ==
  data: x1s input; t1 output; x2s input; lambda1 parameter; lambda2 parameter; max_torque_sagittal parameter; t2 output
% Optimal leg motor torque distribution
function [t1, t2] = distribute_torque(x1s, x2s, lambda1, lambda2, max_torque_sagittal)

s = max_torque_sagittal;

% possible solutions
x1 = [                                                      x1s;
                                                            0;
                                                            s;
                                                            0;
                                                           -s;
  (lambda2*s + lambda1*x1s - lambda2*x2s)/(lambda1 + lambda2);
  (lambda1*x1s - lambda2*s + lambda2*x2s)/(lambda1 + lambda2);
  (lambda2*s + lambda1*x1s + lambda2*x2s)/(lambda1 + lambda2);
 -(lambda2*s - lambda1*x1s + lambda2*x2s)/(lambda1 + lambda2)];
 
x2 = [                                                      x2s;
                                                            s;
                                                            0;
                                                           -s;
                                                            0;
  (lambda1*s - lambda1*x1s + lambda2*x2s)/(lambda1 + lambda2);
  (lambda1*s + lambda1*x1s + lambda2*x2s)/(lambda1 + lambda2);
  (lambda1*x1s - lambda1*s + lambda2*x2s)/(lambda1 + lambda2);
 -(lambda1*s + lambda1*x1s - lambda2*x2s)/(lambda1 + lambda2)];

% test constraints
c1 = s - x1 - x2 >= 0;
c2 = s + x1 + x2 >= 0;
c3 = s - x1 + x2 >= 0;
c4 = s + x1 - x2 >= 0;
constraints = c1 & c2 & c3 & c4;

% objective function to maximize
f = -lambda1*(x1-x1s).^2-lambda2*(x2-x2s).^2;
satisfied = find(constraints);
[~,I] = max(f(satisfied));

t1 = x1(satisfied(I));
t2 = x2(satisfied(I));

== matlab function vertical_smm_with_lqr_2d/Control/Behavior Control/Secondary Leg Behavior/Avoid Hitting Mechanical Limits ==
  data: back_cmd output double; front_cmd output double; dback_cmd output double; dfront_cmd output double; ddback_cmd output double; ddfront_cmd output double; back_desired input; dback_desired input; ddback_desired input; front_desired input; dfront_desired input; ddfront_desired input; min_front_bar_angle parameter; max_front_bar_angle parameter; min_back_bar_angle parameter; max_back_bar_angle parameter
%% Avoid joint limits by ensuring we don't command velocities/accelerations that would push us into them when we are close to them.
function [back_cmd, front_cmd, dback_cmd, dfront_cmd, ddback_cmd, ddfront_cmd] ...
    = AvoidFourbarLimits(back_desired,dback_desired, ddback_desired, ...
          front_desired, dfront_desired, ddfront_desired, ...
          min_front_bar_angle, max_front_bar_angle, min_back_bar_angle, max_back_bar_angle)
    [back_cmd, front_cmd, dback_cmd, dfront_cmd, ddback_cmd, ddfront_cmd] = AvoidFourbarLimits(back_desired,dback_desired, ddback_desired, front_desired, dfront_desired, ddfront_desired, min_front_bar_angle, max_front_bar_angle, min_back_bar_angle, max_back_bar_angle);
end

== matlab function vertical_smm_with_lqr_2d/Control/Behavior Control/State Estimation/PositionUsingRobotGeometry ==
  data: right_left input; horizontal_com_position output; roll input; pitch input; yaw input; horizontal_com_velocity output; lateral_com_position output; lateral_com_velocity output; left_leg_sagittal_angle input; left_leg_lateral_angle input; left_leg_length input; right_leg_sagittal_angle input; right_leg_lateral_angle input; right_leg_length input; m_torso parameter; m_leg_motor parameter; m_leg parameter; com_torso parameter; com_leg_motor parameter; lateral_offset parameter; vertical_com_position output; vertical_com_velocity output; com_left_foot output; dcom_left_foot output; com_right_foot output; dcom_right_foot output; com_pelvis output; dcom_pelvis output
% Returns 2D COM relative to primary foot
function [horizontal_com_position, horizontal_com_velocity, ...
          lateral_com_position, lateral_com_velocity, ...
          vertical_com_position, vertical_com_velocity, ...
          com_left_foot, dcom_left_foot, com_right_foot, dcom_right_foot, ....
          com_pelvis, dcom_pelvis] = ...
         ComPositionUsingRobotGeometry(right_left, ...
                                    roll, pitch, yaw, ...
                                    left_leg_sagittal_angle, left_leg_lateral_angle, left_leg_length, ...
                                    right_leg_sagittal_angle, right_leg_lateral_angle, right_leg_length, ...
                                    m_torso, m_leg_motor, m_leg, com_torso, com_leg_motor, lateral_offset)
                    
    q =  [roll(1), pitch(1), yaw(1), left_leg_sagittal_angle(1), left_leg_lateral_angle(1), left_leg_length(1), right_leg_sagittal_angle(1), right_leg_lateral_angle(1), right_leg_length(1)];
    dq = [roll(2), pitch(2), yaw(2), left_leg_sagittal_angle(2), left_leg_lateral_angle(2), left_leg_length(2), right_leg_sagittal_angle(2), right_leg_lateral_angle(2), right_leg_length(2)];
                    
    [ com_pelvis, dcom_pelvis, ...
      com_left_foot, dcom_left_foot, ...
      com_right_foot, dcom_right_foot ] = ...
    ComCalculationFromRobot( q, dq, m_torso, m_leg_motor, m_leg, com_torso, com_leg_motor, lateral_offset );

    if right_left
        com_position = com_right_foot(4:6);
        com_velocity = dcom_right_foot(4:6);
    else
        com_position = com_left_foot(4:6);
        com_velocity = dcom_left_foot(4:6);
    end


    horizontal_com_position = com_position(1);
    horizontal_com_velocity = com_velocity(1);
    lateral_com_position = com_position(2);
    lateral_com_velocity = com_velocity(2);
    vertical_com_position = com_position(3);
    vertical_com_velocity = com_velocity(3);

end

== matlab function vertical_smm_with_lqr_2d/Control/Behavior Control/Torque Distribution Left/Motor Torque Saturation Optimization ==
  data: x1s input; t1 output; x2s input; lambda1 parameter; lambda2 parameter; max_torque_sagittal parameter; t2 output
% Optimal leg motor torque distribution
function [t1, t2] = distribute_torque(x1s, x2s, lambda1, lambda2, max_torque_sagittal)

s = max_torque_sagittal;

% possible solutions
x1 = [                                                      x1s;
                                                            0;
                                                            s;
                                                            0;
                                                           -s;
  (lambda2*s + lambda1*x1s - lambda2*x2s)/(lambda1 + lambda2);
  (lambda1*x1s - lambda2*s + lambda2*x2s)/(lambda1 + lambda2);
  (lambda2*s + lambda1*x1s + lambda2*x2s)/(lambda1 + lambda2);
 -(lambda2*s - lambda1*x1s + lambda2*x2s)/(lambda1 + lambda2)];
 
x2 = [                                                      x2s;
                                                            s;
                                                            0;
                                                           -s;
                                                            0;
  (lambda1*s - lambda1*x1s + lambda2*x2s)/(lambda1 + lambda2);
  (lambda1*s + lambda1*x1s + lambda2*x2s)/(lambda1 + lambda2);
  (lambda1*x1s - lambda1*s + lambda2*x2s)/(lambda1 + lambda2);
 -(lambda1*s + lambda1*x1s - lambda2*x2s)/(lambda1 + lambda2)];

% test constraints
c1 = s - x1 - x2 >= 0;
c2 = s + x1 + x2 >= 0;
c3 = s - x1 + x2 >= 0;
c4 = s + x1 - x2 >= 0;
constraints = c1 & c2 & c3 & c4;

% objective function to maximize
f = -lambda1*(x1-x1s).^2-lambda2*(x2-x2s).^2;
satisfied = find(constraints);
[~,I] = max(f(satisfied));

t1 = x1(satisfied(I));
t2 = x2(satisfied(I));

== matlab function vertical_smm_with_lqr_2d/Control/Behavior Control/State Estimation/Kalman Filtering/eigen values ==
  data: Z input; E output
function E = eigen(Z)
    E = real(eig(Z));
    E = sort(E);
end

== matlab function vertical_smm_with_lqr_2d/Control/Behavior Control/Primary Leg Behavior/Running/Flight/Generate Parabolic Foot Trajectories ==
  data: time_remaining input; est_duration input; stance input; x_star input; y_star input; x0 input; y0 input; zdz0 input; max_retract input; z_land parameter; min_f_duration parameter; X_star output size=3; Y_star output size=3; Z_star output size=3
%% Parabolic trajectory generation for x, y, and z
% est_duration: estimated flight time
% time_remaining: time until estimated touchdown
% stance: 1 if in stance, 0 otherwise
% x_star: desired x for foot to COM
% y_star: desired y for foot to COM
% x0: x position at takeoff
% y0: y position at takeoff
% zdz0: [z, dz] at takeoff
% max_retract: how high to lift z for ground clearance
% z_land: nominal z height for landing
% min_f_duration: minimum trajectory time

function [X_star, Y_star, Z_star]  =  ...
          GenerateParabolicFootTrajectory(time_remaining, est_duration,  ...
                               stance, x_star, y_star, x0, y0, zdz0, ...
                               max_retract,  z_land, min_f_duration)
% we are solving for yawed coordinates xyz of com-foot in flight and
% converting them to joint angles

% estimate z ballistically
% z = z_dz_liftoff(1) + z_dz_liftoff(2)*t_flight -g/2*t_flight^2;
% dz = z_dz_liftoff(2) - g*t_flight;
% 
% z = com_xdx_ydy_zdz(5); dz = com_xdx_ydy_zdz(6);
% time_remaining = (-dz-sqrt(max(dz^2 - 4*g/2*(z_land-z), 0) ) )/ (-g); % ballistic estimate of landing

% if stance || time_remaining < 0
if stance
  X_star = [0;0;0]; Y_star = [0;0;0]; Z_star = [z_land-max_retract;0;0];   
else
  % plan a traj from init to desired in estimated duration. Use a
  % discontinuous initial condition if estimated duration too short.
  duration = max(est_duration, min_f_duration);
  t_r = max(min(time_remaining, duration),0);
  % sweep a parabola from x0 to x_star with dx_end = 0
  x_star_t = x_star + (x0-x_star)*(t_r/duration)^2;
  dx_star_t = -(x0-x_star)*2*(t_r/duration)/duration;
  ddx_star_t = (x0-x_star)*2/duration^2;
  % same for y
  y_star_t = y_star + (y0-y_star)*(t_r/duration)^2;
  dy_star_t = -(y0-y_star)*2*(t_r/duration)/duration;
  ddy_star_t = (y0-y_star)*2/duration^2;
  
  % split duration into thirds.  First segment: parabola from z0 to
  % max_retract.  Second and third segments, cos to landing.
  z0 = zdz0(1);
  dt3 = duration / 3;
  z_min = z_land - max_retract;
  if t_r > 2*dt3;
    z_star_t = z_min + (z0-z_min)*((t_r-2*dt3)/dt3)^2;
    dz_star_t = -(z0-z_min)*2*(t_r-2*dt3)/dt3/dt3;
    ddz_star_t = (z0-z_min)*2/dt3^2;
  else
    z_star_t = z_land + (z_min-z_land)/2*(1-cos(t_r/(2*dt3)*pi));
    dz_star_t = -(z_min-z_land)/2*sin(t_r/(2*dt3)*pi)*pi/(2*dt3);
    ddz_star_t = (z_min-z_land)/2*cos(t_r/(2*dt3)*pi)*(pi/(2*dt3))^2;
  end
  % track a sinusoidal z of amplitude max_retract, finishing a half-cycle by t_end
  X_star = [x_star_t; dx_star_t; ddx_star_t];
  Y_star = [y_star_t; dy_star_t; ddy_star_t];
  Z_star = [z_star_t; dz_star_t; ddz_star_t];
end

== matlab function vertical_smm_with_lqr_2d/Control/Behavior Control/Primary Leg Behavior/Running/Stance/LQR Feedback for Desired Vertical GRF ==
  data: hopping input; stance input; zdzddz_ref input size=3; GRFz_desired output; z_state input; leg_length input; k_LQR_vertical parameter; P_LQR_vertical parameter; k_vertical_winch parameter; m_total_real parameter; g parameter; cost_to_go output double size=1; max_leg_length parameter
%% LQR for z during stance

% stance: 1 if in stance, 0 otherwise
% z_state: [z, dz] current estimate
% zdzddz_ref: reference trajectory for z position, velocity, and acceleration


% GRFz_desired: desired z GRF
% cost_to_go: remaining LQR cost

function [GRFz_desired, cost_to_go]   =  ...
               LQR_Vertical_Height(hopping, stance, zdzddz_ref, z_state, leg_length,...
                                   k_LQR_vertical, P_LQR_vertical, k_vertical_winch, m_total_real, g, max_leg_length)

    z_ref = zdzddz_ref(1:2);     
    ddz_ref = zdzddz_ref(3);
    z_error = (z_state - z_ref);
    GRFz_desired = m_total_real*(g+ddz_ref) - k_LQR_vertical*z_error;
    
    if z_ref(2) < 0
      GRFz_desired = max(50, GRFz_desired);
    end
    
    % Prevent leg over extentsion
    if leg_length(1) >= max_leg_length - 0.025
        GRFz_desired = 0;
    end
    
    if ~hopping
        GRFz_desired = m_total_real*g - k_vertical_winch*z_error;
        GRFz_desired = max(200, GRFz_desired);
    end
    
    
    
    cost_to_go = z_error'*P_LQR_vertical*z_error;
    
    if stance == 0
      GRFz_desired = 0;
      cost_to_go = 0;
    end
end

== matlab function vertical_smm_with_lqr_2d/Control/Behavior Control/Primary Leg Behavior/Running/Circular Buffer/Buffer6 ==
  data: data input; buffer output size=recorded_steps; trigger input; buffer_size input
function buffer  = buffer_data(data, trigger, buffer_size)

    persistent buffer_memory
    coder.varsize('buffer_memory',100);
    if isempty(buffer_memory)
        buffer_memory = [];
    end
    
    if trigger
        buffer_memory = [data; buffer_memory];
        if size(buffer_memory, 1) > buffer_size
            buffer_memory = buffer_memory(1:buffer_size,:);
        end
    end
    
    buffer = buffer_memory;

end
